simulink model "simulink_control"  (R2020a)
settings: Solver=ode1  StartTime=0.0  StopTime=10.0  FixedStep=0.01  RelTol=1e-3
libraries: robotlib x8
settings Model: Creator=Steph  LastModifiedBy=mahsa
settings OptimizationCC: EnhancedBackFolding=on  PassReuseOutputArgsAs=Individual arguments  ZeroExternalMemoryAtStartup=off  ZeroInternalMemoryAtStartup=off  MaxStackSize=64  OptimizeBlockOrder=speed  DifferentSizesBufferReuse=on  OptimizationCustomize=off  EfficientTunableParamExpr=on
settings DebuggingCC: ParameterTunabilityLossMsg=error
settings HardwareCC: ProdBitPerPointer=32  ProdBitPerSizeT=32  ProdBitPerPtrDiffT=32  ProdLargestAtomicFloat=None  ProdIntDivRoundTo=Undefined  ProdEndianess=Unspecified  ProdWordSize=32  ProdHWDeviceType=Generic->Unspecified (assume 32-bit Generic)
settings SFSimCC: MATLABDynamicMemAlloc=off
settings RTWCC: SystemTargetFile=ert.tlc  HardwareBoard=Robot Operating System (ROS)  TemplateMakefile=ert_default_tmf  GenerateReport=on  Toolchain=Catkin  IncludeHyperlinkInReport=on  LaunchReport=on  TargetLang=C++  GenerateTraceInfo=on  GenerateTraceReport=on  GenerateTraceReportSl=on  GenerateTraceReportSf=on  GenerateTraceReportEml=on
settings CodeAppCC: ForceParamTrailComments=on  IgnoreCustomStorageClasses=off  OperatorAnnotations=on  SimulinkDataObjDesc=on  SFDataObjDesc=on  InsertBlockDesc=on
settings ERTTargetCC: SupportContinuousTime=on  SupportVariableSizeSignals=on

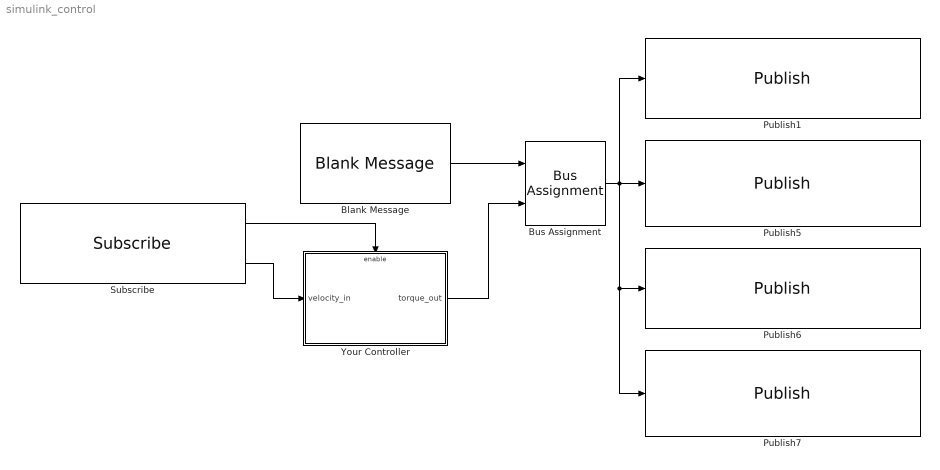
== system simulink_control ==
  Blank Message : robotlib/Blank Message  messageClass=Message  entityType=std_msgs/Float64  messageType=std_msgs/Float64  SampleTime=inf
  Bus Assignment : BusAssignment  AssignedSignals=Data
  Publish1 : robotlib/Publish  topicSource=Specify your own  topic=/racecar/internal/left_front_controller/command  messageType=std_msgs/Float64  messageQueueLength=1
  Publish5 : robotlib/Publish  topicSource=Specify your own  topic=/racecar/internal/left_rear_controller/command  messageType=std_msgs/Float64  messageQueueLength=1
  Publish6 : robotlib/Publish  topicSource=Specify your own  topic=/racecar/internal/right_front_controller/command  messageType=std_msgs/Float64  messageQueueLength=1
  Publish7 : robotlib/Publish  topicSource=Specify your own  topic=/racecar/internal/left_rear_controller/command  messageType=std_msgs/Float64  messageQueueLength=1
  Subscribe : robotlib/Subscribe  topicSource=Specify your own  topic=/racecar/internal/sim_only/global_pos  messageType=nav_msgs/Odometry  sampleTime=-1  messageQueueLength=1
  Your Controller : Subsystem
  wires:
  Your Controller/1(torque_out) -> Bus Assignment/2
  Blank Message/1 -> Bus Assignment/1
  Bus Assignment/1 -> Publish7/1, Publish6/1, Publish5/1, Publish1/1
  Subscribe/2 -> Your Controller/1(velocity_in)
  Subscribe/1 -> Your Controller/Enable

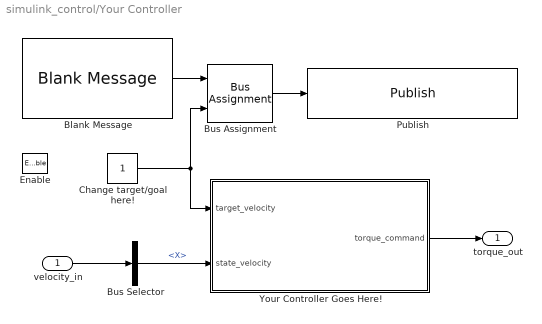
== system simulink_control/Your Controller ==
  velocity_in : Inport
  Enable : EnablePort
  Blank Message : robotlib/Blank Message  messageClass=Message  entityType=std_msgs/Float64  messageType=std_msgs/Float64  SampleTime=inf
  Bus Assignment : BusAssignment  AssignedSignals=Data
  Bus Selector : BusSelector  OutputSignals=Twist.Twist.Linear.X
  Change target/goal here! : Constant
  Publish : robotlib/Publish  topicSource=Specify your own  topic=/racecar/internal/long_control_target  messageType=std_msgs/Float64  messageQueueLength=1
  Your Controller Goes Here! : MATLAB Function  TreatAsAtomicUnit=on
  torque_out : Outport
  wires:
  velocity_in/1 -> Bus Selector/1
  Bus Selector/1 -> Your Controller Goes Here!/2(state_velocity)  "<X>"
  Change target/goal here!/1 -> Bus Assignment/2, Your Controller Goes Here!/1(target_velocity)
  Your Controller Goes Here!/1(torque_command) -> torque_out/1
  Blank Message/1 -> Bus Assignment/1
  Bus Assignment/1 -> Publish/1

== matlab function simulink_control/Your Controller/Your Controller Goes Here! ==
  data: target_velocity input; torque_command output; state_velocity input
function torque_command = compute_control(target_velocity, state_velocity)
% feel free to swap out this block for another one when permitted
torque_command = (target_velocity - state_velocity) * 4.5;
